simulink model "CIM_MBCD"  (R2016b)
settings: Solver=FixedStepDiscrete  StartTime=0.0  StopTime=500  FixedStep=TimeSteps.ModelStep  RelTol=1e-3
libraries: FMIKit_blocks x1
settings Model: Creator=KIRTACA  LastModifiedBy=KIRTACA

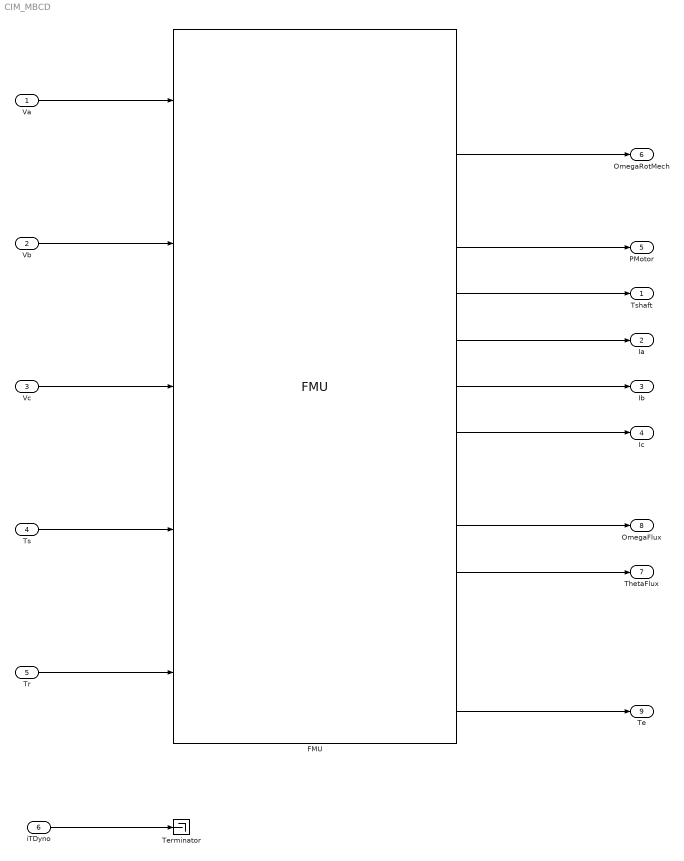
== system CIM_MBCD ==
  Va : Inport
  Vb : Inport  Port=2
  Vc : Inport  Port=3
  Ts : Inport  Port=4
  Tr : Inport  Port=5
  iTDyno : Inport  Port=6
  FMU : FMIKit_blocks/FMU
  Terminator : Terminator
  Tshaft : Outport
  Ia : Outport  Port=2
  Ib : Outport  Port=3
  Ic : Outport  Port=4
  PMotor : Outport  Port=5
  OmegaRotMech : Outport  Port=6
  ThetaFlux : Outport  Port=7
  OmegaFlux : Outport  Port=8
  Te : Outport  Port=9
  wires:
  FMU/3 -> OmegaRotMech/1
  FMU/5 -> PMotor/1
  FMU/6 -> Tshaft/1
  FMU/7 -> Ia/1
  FMU/8 -> Ib/1
  FMU/9 -> Ic/1
  FMU/11 -> OmegaFlux/1
  FMU/12 -> ThetaFlux/1
  iTDyno/1 -> Terminator/1
  Va/1 -> FMU/1
  Vb/1 -> FMU/2
  Vc/1 -> FMU/3
  Tr/1 -> FMU/5
  Ts/1 -> FMU/4
  FMU/15 -> Te/1
